simulink library "VANETlib"  (R2019b)
settings: Solver=VariableStepAuto  StartTime=0.0  StopTime=10.0  RelTol=1e-3
PreLoadFcn:
  | vanet_init();
StartFcn:
  | vanet_init();
undefined symbols (not defined in the file or in its folder): fcn_initInfo, m
libraries: $bdroot x2
settings Model: Creator=Le  LastModifiedBy=lewang
settings DataIOCC: ReturnWorkspaceOutputs=off
settings DebuggingCC: ArithmeticOperatorsInVariantConditions=warning
settings SFSimCC: SimUseLocalCustomCode=off  CustomCodeUndefinedFunction=UseInterfaceOnly
settings RTWCC: RTWUseLocalCustomCode=off
settings CodeAppCC: StateflowObjectComments=on

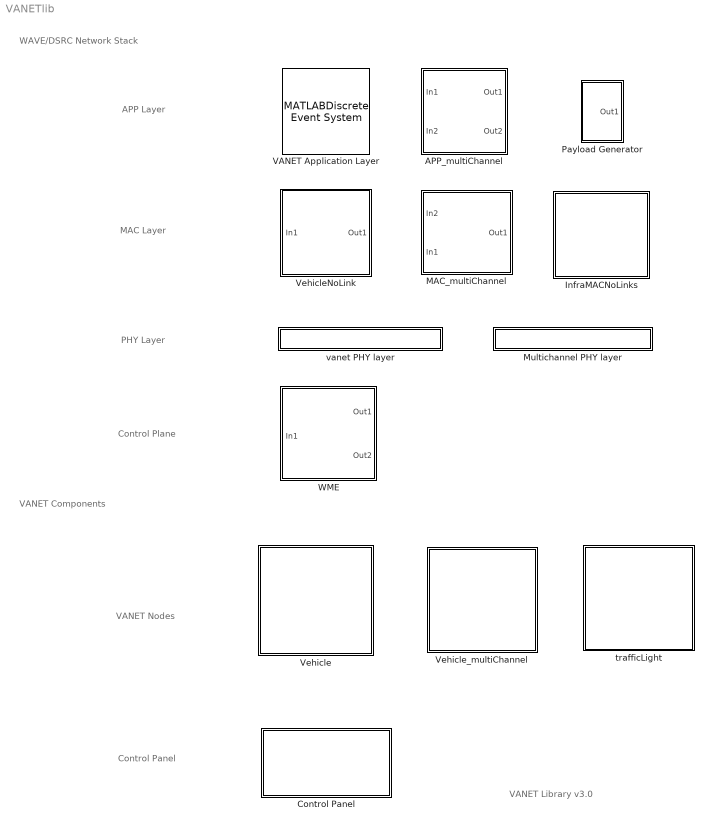
== system VANETlib ==
  note: VANET Components
  note: WAVE/DSRC Network Stack
  note: VANET Library v3.0
  note: APP Layer
  note: MAC Layer
  note: PHY Layer
  note: VANET Nodes
  note: Control Panel
  note: Control Plane
  APP_multiChannel : Subsystem  mask{vehicleID=1, initVelocity=50, initAcc=10, initLane=1, startPositionX=100, startPositionY=0}
      mask prompts: vehicleID "Vehicle ID:"; initVelocity "Start Speed(km/h):"; initAcc "Seconds (0 - 100km/h):"; initLane "Initial Lane (1-4):"; startPositionX "Initial PositionX:"; startPositionY "Initial PositionY:"
      mask Display:
      | str = sprintf('%s\n%s', 'APP', '(Multi-Channel)');
      | disp(str);
  Control Panel : Subsystem  StartFcn=fcn_initInfo('init');  mask{road=highway, roadLength=1600, speedLimit=60, laneChangingOption=Brake without Lane Changing, emgLaneChangingOption=EMG Brake without Lane Changing, txtEnable=off, appTXTEnable=off, isUIon=on, enCCHIext=off}
      mask prompts: road "Road Type"; roadLength "Length of the road (meters)"; speedLimit "Speed limit (km/h)"; laneChangingOption "Lane Changing Option"; emgLaneChangingOption "EMG Lane Changing Option"; txtEnable "Show MAC_PHY Text Process"; appTXTEnable "Show APP Text Process"; isUIon "Graphic UI"; enCCHIext "Enable CCHI_Extension"
      mask init:
      | evalin('base',['txtEnable=' num2str(txtEnable) ';']);
      | evalin('base',['appTXTEnable=' num2str(appTXTEnable) ';']);
      | evalin('base',['roadLength=' num2str(roadLength) ';']);
      | evalin('base',['speedLimit=' num2str(speedLimit) ';']);
      | evalin('base',['isUIon=' num2str(isUIon) ';']);
      | evalin('base',['enCCHIext=' num2str(enCCHIext) ';']);
      mask TypeOptions road: highway | crossRD
      mask Callback road:
      | r=get_param(gcb,'road');
      | assignin('base','road',r);
      mask TypeOptions laneChangingOption: Conservative Lane Changing | Performance Lane Changing | Brake without Lane Changing
      mask Callback laneChangingOption:
      | str=get_param(gcb,'laneChangingOption');
      | 
      | if strcmp(str(1),'C')
      |     assignin('base','brakeMode','ConLaneChange');
      | elseif strcmp(str(1),'P')
      |     assignin('base','brakeMode','PerLaneChange');
      | else
      |     assignin('base','brakeMode','NonLaneChange');
      | end
      mask TypeOptions emgLaneChangingOption: Conservative EMG Lane Changing | Performance EMG Lane Changing | EMG Brake without Lane Changing
      mask Display:
      | str=sprintf('%s\n%s','Parameter','Control Panel');
      | disp(str);
  InfraMACNoLinks : Subsystem
      mask Display:
      | str=sprintf('%s\n%s','InfrastructureMAC','(RoadSideUnit)');
      | disp(str);
  "MAC_multiChannel " : Subsystem  mask{txAddr=0}
      mask prompts: txAddr "Vehicle ID"
      mask Display:
      | str = sprintf('%s\n%s', 'VehicleMAC','(Multi-Channel)');
      | disp(str);
  Multichannel PHY layer : Subsystem  mask{numStations=4}
      mask prompts: numStations "Number of vehicles"
      mask init:
      | evalin('base',['numStations=' num2str(numStations) ';']);
      mask Display: disp('Wireless MultiChannel');
  Payload Generator : Subsystem  mask{txAddr=1, ac0Rate=1, ac1Rate=1, ac2Rate=1, ac3Rate=1}
      mask prompts: txAddr "StationID"; ac0Rate "AC0"; ac1Rate "AC1"; ac2Rate "AC2"; ac3Rate "AC3"
      mask Display: disp('msg');
  VANET Application Layer : MATLABDiscreteEventSystem  InputPortMessageModes=m  OutputPortMessageModes=m  System=des_APP_OBU  vehicleID=1  initVelocity=10  initAcc=10  initLane=1  startPositionX=10  startPositionY=0  SimulateUsing=Code generation
      mask Type: des_APP_OBU
      mask Display: disp('des_APP_OBU');
  Vehicle : Subsystem  mask{carID=1, startSpd=50, startAcc=10, initLane=1, startPosX=0, startPosY=0}
      mask prompts: carID "VehilcleID"; startSpd "Initial Speed (Km/h):"; startAcc "Seconds from 0 - 100 Km/h:"; initLane "Initial lane number (1-4) :"; startPosX "Initial PositionX"; startPosY "Initial PositionY"
      mask Display:
      | str=sprintf('%s\n%s','Vehicle','(APP-MAC-PHY)');
      | disp(str);
      | 
      | image('figs/car2.jpg');
  VehicleNoLink : Subsystem  mask{txAddr=1, V2x=V2V, infraAddress=0, Retry_MAX=3, AC0=9, AC1=6, AC2=3, AC3=2, aCWmin=15, aCWmax=1023, slottime=13, SIFS=32}
      mask prompts: txAddr "Vehicle ID"; V2x "V2X Mode"; infraAddress "AP"; Retry_MAX "Max Retransmissions (3-8):"; AC0 "AIFSN(AC0):"; AC1 "AIFSN(AC1):"; AC2 "AIFSN(AC2):"; AC3 "AIFSN(AC3):"; slottime "slotTime (us):"; SIFS "SIFS (us):"
      mask TypeOptions V2x: V2V | V2I
      mask Callback V2x:
      | V2Xmode=get_param(gcb,'V2x');
      | 
      | if strcmp(V2Xmode,'V2V')
      |     set_param(gcb,'MaskVisibilities',{'on';'on';'off';'on';'on';'on';'on';'on';'on';'on';'on';'on'});
      | 
      | elseif strcmp(V2Xmode,'V2I')
      |     set_param(gcb,'MaskVisibilities',{'on';'on';'on';'on';'on';'on';'on';'on';'on';'on';'on';'on'});
      | end
      mask DialogControl netParams Prompt: Network Parameters
      mask DialogControl Basic Prompt: Basic Information
      mask DialogControl EDCA Prompt: EDCA Parameter
      mask Display:
      | str=sprintf('%s\n%s','VehicleMAC','(OnBoardUnit)');
      | disp(str);
  Vehicle_multiChannel : Subsystem  mask{vehicleID=1, startSpd=50, startAcc=10, initLane=1, startPosX=100, startPosY=0, MCsvcRole=Service User}
      mask prompts: vehicleID "Vehicle ID"; startSpd "Initial Speed(km/h):"; startAcc "Seconds from 0-100 km/h:"; initLane "Initial lane number(1-4):"; startPosX "Initial PositionX:"; startPosY "Initial PositionY:"; MCsvcRole "Service Role (Provider/User):"
      mask TypeOptions MCsvcRole: Service Provider | Service User
      mask Callback MCsvcRole: MCsvcRole=get_param(gcb,'MCsvcRole');
      mask Display:
      | %disp('vehicle_multiChan');
      | 
      | image('figs/car2.png');
  WME : Subsystem  mask{vehicleID=1}
      mask prompts: vehicleID "Vehicle ID"
      mask Display:
      | str = sprintf('%s\n\n%s\n\n%s\n\n%s', 'WAVE', 'Management', 'Entity', '(WME)');
      | disp(str);
  trafficLight : Subsystem  mask{green=26, yellow=4}
      mask prompts: green "Green Light Duration"; yellow "Yellow Light Duration"
      mask Display:
      | str=sprintf('%s','Traffic Light');
      | disp(str);
      | 
      | image('figs/light2.jpg');
  vanet PHY layer : Subsystem  mask{numStations=0}
      mask prompts: numStations "Number of Vehicles"
      mask init:
      | evalin('base',['numStations=' num2str(numStations) ';']);
      mask Display:
      | disp('Wireless Channel');
      | % image('figs/wave1.png');

== system VANETlib/APP_multiChannel ==
  In1 : Inport
  In2 : Inport  Port=2
  MATLAB Discrete-Event System : MATLABDiscreteEventSystem  InputPortMessageModes=m,m  OutputPortMessageModes=m,m  System=des_APP_mulChan_OBU  vehicleID=vehicleID  initVelocity=initVelocity  initAcc=initAcc  initLane=initLane  startPositionX=startPositionX  startPositionY=startPositionY  svcRole=0  SimulateUsing=Code generation
      mask Type: des_APP_mulChan_OBU
      mask Display: disp('des_APP_mulChan_OBU');
  Out1 : Outport  VectorParamsAs1DForOutWhenUnconnected=off
  Out2 : Outport  Port=2  VectorParamsAs1DForOutWhenUnconnected=off
  wires:
  MATLAB Discrete-Event System/2 -> Out2/1
  In1/1 -> MATLAB Discrete-Event System/1
  In2/1 -> MATLAB Discrete-Event System/2
  MATLAB Discrete-Event System/1 -> Out1/1

== system VANETlib/Control Panel ==

== system VANETlib/InfraMACNoLinks ==
  Entity Multicast : EntityMulticast  InputPortMessageModes=m  MulticastTag=toPhy
  MATLAB Discrete-Event System : MATLABDiscreteEventSystem  InputPortMessageModes=m  OutputPortMessageModes=m  System=des_MAC_RSU  Retry_MAX=3  AIFSN_AC0=9  AIFSN_AC1=6  AIFSN_AC2=3  AIFSN_AC3=2  aCWmin=15  aCWmax=1023  slottime=0.000013  sifs=0.000032  propTime=1  BSSID=00  rxAddr=0  SimulateUsing=Code generation
      mask Type: des_MAC_RSU
      mask Display: disp('des_MAC_RSU');
  Multicast Receive Queue : Queue  OutputPortMessageModes=m  Capacity=inf  EntityArrivalSource=Multicast  MulticastTag=fromPhy
  wires:
  Multicast Receive Queue/1 -> MATLAB Discrete-Event System/1
  MATLAB Discrete-Event System/1 -> Entity Multicast/1

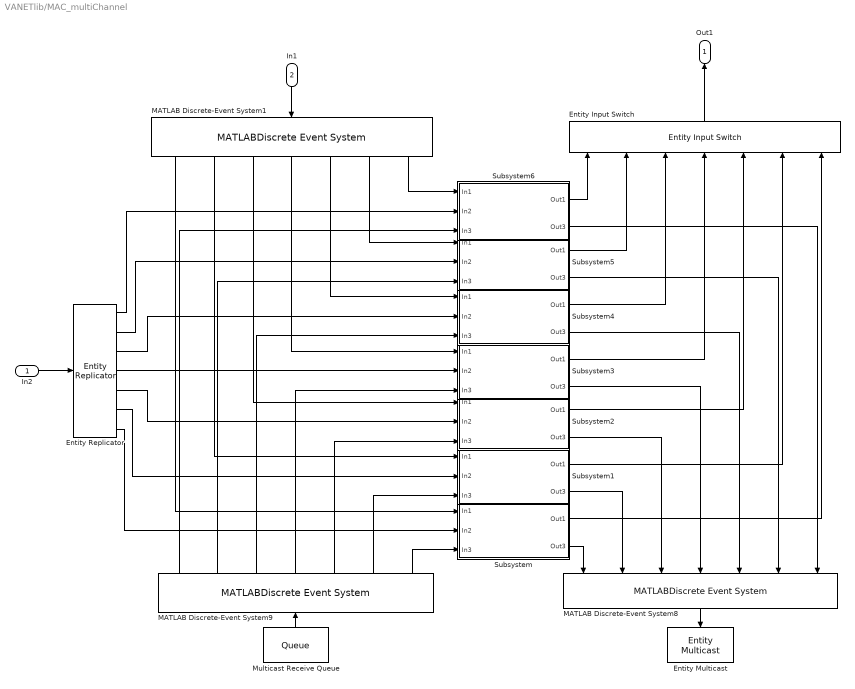
== system VANETlib/MAC_multiChannel  ==
  In2 : Inport
  In1 : Inport  Port=2
  Entity Input Switch : EntityInputSwitch  InputPortMessageModes=m,m,m,m,m,m,m  OutputPortMessageModes=m  NumberInputPorts=7  SwitchingCriterion=Equiprobable
      settings: InputPortMap=u1,u2,u3,u4,u5,u6,u7
  Entity Multicast : EntityMulticast  InputPortMessageModes=m  MulticastTag=toPhy
  Entity Replicator : EntityReplicator  InputPortMessageModes=m  OutputPortMessageModes=m,m,m,m,m,m,m  NumberReplicas=6
      settings: OutputPortMap=o0,o1,o2,o3,o4,o5,o6
  MATLAB Discrete-Event System1 : MATLABDiscreteEventSystem  InputPortMessageModes=m  OutputPortMessageModes=m,m,m,m,m,m,m  System=des_MAC_channelRouting  SimulateUsing=Code generation
      mask Type: des_MAC_channelRouting
      mask Display: disp('des_MAC_channelRouting');
  MATLAB Discrete-Event System8 : MATLABDiscreteEventSystem  InputPortMessageModes=m,m,m,m,m,m,m  OutputPortMessageModes=m  System=des_MAC_channelSelect  SimulateUsing=Code generation
      mask Type: des_MAC_channelSelect
      mask Display: disp('des_MAC_channelSelect');
  MATLAB Discrete-Event System9 : MATLABDiscreteEventSystem  InputPortMessageModes=m  OutputPortMessageModes=m,m,m,m,m,m,m  System=des_MAC_macSelect  SimulateUsing=Code generation
      mask Type: des_MAC_macSelect
      mask Display: disp('des_MAC_macSelect');
  Multicast Receive Queue : Queue  OutputPortMessageModes=m  Capacity=inf  EntityArrivalSource=Multicast  MulticastTag=fromPhy
  Subsystem : Subsystem  mask{chanNum=0}
      mask prompts: chanNum "Channel Number (CCH - 0) :"
      mask Display: disp('CCH - 0');
  Subsystem1 : Subsystem  mask{chanNum=1}
      mask prompts: chanNum "Channel Num (SCH (1-6)):"
      mask Display: disp('SCH - 1');
  Subsystem2 : Subsystem  mask{chanNum=2}
      mask prompts: chanNum "Channel Number (SCH (1-6)) :"
      mask Display: disp('SCH - 2');
  Subsystem3 : Subsystem  mask{chanNum=3}
      mask prompts: chanNum "Channel Number (SCH (1-6)):"
      mask Display: disp('SCH - 3');
  Subsystem4 : Subsystem  mask{chanNum=4}
      mask prompts: chanNum "Channel Number (SCH (1-6)):"
      mask Display: disp('SCH - 4');
  Subsystem5 : Subsystem  mask{chanNum=5}
      mask prompts: chanNum "Channel Number (SCH (1-6)):"
      mask Display: disp('SCH - 5');
  Subsystem6 : Subsystem  mask{chanNum=6}
      mask prompts: chanNum "Channel Number (SCH (1-6)):"
      mask Display: disp('SCH - 6');
  Out1 : Outport  VectorParamsAs1DForOutWhenUnconnected=off
  wires:
  Subsystem3/2(Out3) -> MATLAB Discrete-Event System8/4
  Entity Replicator/7 -> Subsystem/2(In2)
  Subsystem5/2(Out3) -> MATLAB Discrete-Event System8/6
  MATLAB Discrete-Event System9/7 -> Subsystem/3(In3)
  Entity Replicator/5 -> Subsystem2/2(In2)
  MATLAB Discrete-Event System1/7 -> Subsystem6/1(In1)
  Entity Replicator/4 -> Subsystem3/2(In2)
  MATLAB Discrete-Event System1/3 -> Subsystem2/1(In1)
  Subsystem6/1(Out1) -> Entity Input Switch/1
  MATLAB Discrete-Event System9/4 -> Subsystem3/3(In3)
  Subsystem4/2(Out3) -> MATLAB Discrete-Event System8/5
  MATLAB Discrete-Event System9/6 -> Subsystem1/3(In3)
  Subsystem1/2(Out3) -> MATLAB Discrete-Event System8/2
  MATLAB Discrete-Event System1/1 -> Subsystem/1(In1)
  Subsystem/1(Out1) -> Entity Input Switch/7
  Entity Replicator/3 -> Subsystem4/2(In2)
  MATLAB Discrete-Event System9/1 -> Subsystem6/3(In3)
  In2/1 -> Entity Replicator/1
  MATLAB Discrete-Event System1/6 -> Subsystem5/1(In1)
  Subsystem2/2(Out3) -> MATLAB Discrete-Event System8/3
  MATLAB Discrete-Event System8/1 -> Entity Multicast/1
  MATLAB Discrete-Event System9/5 -> Subsystem2/3(In3)
  MATLAB Discrete-Event System9/2 -> Subsystem5/3(In3)
  Subsystem3/1(Out1) -> Entity Input Switch/4
  Subsystem2/1(Out1) -> Entity Input Switch/5
  MATLAB Discrete-Event System9/3 -> Subsystem4/3(In3)
  Subsystem5/1(Out1) -> Entity Input Switch/2
  Entity Input Switch/1 -> Out1/1
  Subsystem1/1(Out1) -> Entity Input Switch/6
  MATLAB Discrete-Event System1/2 -> Subsystem1/1(In1)
  Subsystem6/2(Out3) -> MATLAB Discrete-Event System8/7
  MATLAB Discrete-Event System1/4 -> Subsystem3/1(In1)
  In1/1 -> MATLAB Discrete-Event System1/1
  MATLAB Discrete-Event System1/5 -> Subsystem4/1(In1)
  Subsystem4/1(Out1) -> Entity Input Switch/3
  Entity Replicator/2 -> Subsystem5/2(In2)
  Subsystem/2(Out3) -> MATLAB Discrete-Event System8/1
  Multicast Receive Queue/1 -> MATLAB Discrete-Event System9/1
  Entity Replicator/6 -> Subsystem1/2(In2)
  Entity Replicator/1 -> Subsystem6/2(In2)

== system VANETlib/Multichannel PHY layer ==
  Entity Multicast2 : EntityMulticast  InputPortMessageModes=m  MulticastTag=fromPhy
  MATLAB Discrete-Event System : MATLABDiscreteEventSystem  InputPortMessageModes=m  OutputPortMessageModes=m  System=des_PHY_mulChan_links  SimulateUsing=Code generation
      mask Type: des_PHY_mulChan_links
      mask Display: disp('des_PHY_mulChan_links');
  Multicast Receive Queue2 : Queue  OutputPortMessageModes=m  Capacity=inf  EntityArrivalSource=Multicast  MulticastTag=toPhy
  wires:
  Multicast Receive Queue2/1 -> MATLAB Discrete-Event System/1
  MATLAB Discrete-Event System/1 -> Entity Multicast2/1

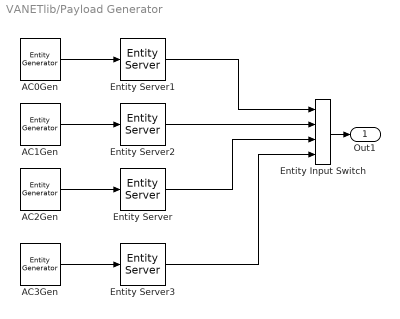
== system VANETlib/Payload Generator ==
  AC0Gen : EntityGenerator  OutputPortMessageModes=m  TimeSource=MATLAB action  Period=0.1  IntergenerationTimeAction=|  GenerateEntityAtSimulationStart=off  GenerateAction=|  EntityType=Bus object  EntityTypeName=Payload
      IntergenerationTimeAction=|
      | % y=getParams();
      | dt=ac0Rate;
      GenerateAction=|
      | coder.extrinsic('evalin')
      | payloadlength=evalin('base','payloadLength');
      | entity.wsmp=ones(1,payloadlength);
      | % rng('shuffle');
      | entity.priority=1;
  AC1Gen : EntityGenerator  OutputPortMessageModes=m  TimeSource=MATLAB action  Period=0.1  IntergenerationTimeAction=|  GenerateEntityAtSimulationStart=off  GenerateAction=|  EntityType=Bus object  EntityTypeName=Payload
      IntergenerationTimeAction=|
      | % y=getParams();
      | dt=ac1Rate;
      GenerateAction=|
      | coder.extrinsic('evalin')
      | payloadlength=evalin('base','payloadLength');
      | entity.wsmp=ones(1,payloadlength);
      | % rng('shuffle');
      | entity.priority=3;
  AC2Gen : EntityGenerator  OutputPortMessageModes=m  TimeSource=MATLAB action  Period=0.1  IntergenerationTimeAction=|  GenerateEntityAtSimulationStart=off  GenerateAction=|  EntityType=Bus object  EntityTypeName=Payload
      IntergenerationTimeAction=|
      | % y=getParams();
      | dt=ac2Rate;
      GenerateAction=|
      | coder.extrinsic('evalin')
      | payloadlength=evalin('base','payloadLength');
      | entity.wsmp=ones(1,payloadlength);
      | entity.VehicleID=txAddr;
      | % rng('shuffle');
      | entity.priority=5;
  AC3Gen : EntityGenerator  OutputPortMessageModes=m  TimeSource=MATLAB action  Period=0.1  IntergenerationTimeAction=|  GenerateEntityAtSimulationStart=off  GenerateAction=|  EntityType=Bus object  EntityTypeName=Payload
      IntergenerationTimeAction=|
      | % dt=exponentialArrivalTime();
      | dt=ac3Rate;
      GenerateAction=|
      | coder.extrinsic('evalin')
      | payloadLength=evalin('base','payloadLength');
      | entity.wsmp=ones(1,payloadLength);
      | 
      | % entity.wsmp=msg2wsmp(txAddr,entity.wsmp,1);
      | % rng('shuffle');
      | entity.priority=7;
  Entity Input Switch : EntityInputSwitch  InputPortMessageModes=m,m,m,m  OutputPortMessageModes=m  NumberInputPorts=4
      settings: InputPortMap=u1,u2,u3,u4
  Entity Server : EntityServer  InputPortMessageModes=m  OutputPortMessageModes=m  Capacity=1  ServiceTimeSource=MATLAB action  ServiceTimeAction=dt = 0.000002*txAddr;
  Entity Server1 : EntityServer  InputPortMessageModes=m  OutputPortMessageModes=m  Capacity=1  ServiceTimeSource=MATLAB action  ServiceTimeAction=dt = 0.000004*txAddr;
  Entity Server2 : EntityServer  InputPortMessageModes=m  OutputPortMessageModes=m  Capacity=1  ServiceTimeSource=MATLAB action  ServiceTimeAction=dt = 0.000003*txAddr;
  Entity Server3 : EntityServer  InputPortMessageModes=m  OutputPortMessageModes=m  Capacity=1  ServiceTimeSource=MATLAB action  ServiceTimeAction=dt = 0.000001*txAddr;
  Out1 : Outport  VectorParamsAs1DForOutWhenUnconnected=off
  wires:
  AC2Gen/1 -> Entity Server/1
  Entity Server/1 -> Entity Input Switch/3
  Entity Input Switch/1 -> Out1/1
  AC0Gen/1 -> Entity Server1/1
  Entity Server1/1 -> Entity Input Switch/1
  AC1Gen/1 -> Entity Server2/1
  Entity Server2/1 -> Entity Input Switch/2
  AC3Gen/1 -> Entity Server3/1
  Entity Server3/1 -> Entity Input Switch/4

== system VANETlib/Vehicle ==
  VANET Application Layer1 : $bdroot/VANET Application Layer  vehicleID=carID  initVelocity=startSpd  initAcc=startAcc  initLane=initLane  startPositionX=startPosX  startPositionY=startPosY  SimulateUsing=Code generation
  VehicleOI1 : $bdroot/VehicleNoLink  txAddr=carID  V2x=V2V  infraAddress=0  Retry_MAX=3  AC0=9  AC1=6  AC2=3  AC3=2  aCWmin=15  aCWmax=1023  slottime=13  SIFS=32
  wires:
  VehicleOI1/1 -> VANET Application Layer1/1
  VANET Application Layer1/1 -> VehicleOI1/1

== system VANETlib/VehicleNoLink ==
  In1 : Inport
  Entity Multicast : EntityMulticast  InputPortMessageModes=m  MulticastTag=toPhy
  Multicast Receive Queue : Queue  OutputPortMessageModes=m  Capacity=inf  EntityArrivalSource=Multicast  MulticastTag=fromPhy
  vehicular OBU : MATLABDiscreteEventSystem  InputPortMessageModes=m,m  OutputPortMessageModes=m,m  System=des_MAC_OBU  Retry_MAX=Retry_MAX  AIFSN_AC0=AC0  AIFSN_AC1=AC1  AIFSN_AC2=AC2  AIFSN_AC3=AC3  aCWmin=aCWmin  aCWmax=aCWmax  slottime=slottime  sifs=SIFS  txAddr=txAddr  infraAddress=infraAddress  SimulateUsing=Code generation
      mask Type: des_MAC_OBU
      mask Display: disp('des_MAC_OBU');
  Out1 : Outport  VectorParamsAs1DForOutWhenUnconnected=off
  wires:
  In1/1 -> vehicular OBU/1
  vehicular OBU/1 -> Out1/1
  Multicast Receive Queue/1 -> vehicular OBU/2
  vehicular OBU/2 -> Entity Multicast/1

== system VANETlib/Vehicle_multiChannel ==
  MATLAB Discrete-Event System1 : MATLABDiscreteEventSystem  InputPortMessageModes=m,m  OutputPortMessageModes=m,m  System=des_APP_mulChan_OBU  vehicleID=vehicleID  initVelocity=startSpd  initAcc=startAcc  initLane=initLane  startPositionX=startPosX  startPositionY=startPosY  svcRole=0  SimulateUsing=Code generation
      mask Type: des_APP_mulChan_OBU
      mask Display: disp('des_APP_mulChan_OBU');
  Subsystem1 : Subsystem  mask{txAddr=vehicleID}
      mask prompts: txAddr "Vehicle ID"
      mask Display: disp('des_MAC_mulChan_OBU');
  Subsystem2 : Subsystem  mask{vehicleID=vehicleID}
      mask prompts: vehicleID "Vehicle ID"
      mask Display:
      | str = sprintf('%s\n\n%s\n\n%s\n\n%s', 'WAVE', 'Management', 'Entity', '(WME)');
      | disp(str);
  wires:
  Subsystem2/2(Out2) -> Subsystem1/1(In2)
  MATLAB Discrete-Event System1/1 -> Subsystem1/2(In1)
  Subsystem1/1(Out1) -> MATLAB Discrete-Event System1/1
  Subsystem2/1(Out1) -> MATLAB Discrete-Event System1/2
  MATLAB Discrete-Event System1/2 -> Subsystem2/1(In1)

== system VANETlib/WME ==
  In1 : Inport
  MATLAB Discrete-Event System : MATLABDiscreteEventSystem  InputPortMessageModes=m  OutputPortMessageModes=m,m  System=des_APP_WME  vehicleID=0  enCCHIext=0  SimulateUsing=Code generation
      mask Type: des_APP_WME
      mask Display: disp('des_APP_WME');
  Out1 : Outport  VectorParamsAs1DForOutWhenUnconnected=off
  Out2 : Outport  Port=2  VectorParamsAs1DForOutWhenUnconnected=off
  wires:
  MATLAB Discrete-Event System/1 -> Out1/1
  In1/1 -> MATLAB Discrete-Event System/1
  MATLAB Discrete-Event System/2 -> Out2/1

== system VANETlib/trafficLight ==
  Entity Generator : EntityGenerator  OutputPortMessageModes=m  Period=inf  GenerateAction=|  AttributeName=entity  AttributeInitialValue=0  EntityTypeName=Entity
      | persistent n
      | if isempty(n)
      |     n=1;
      | end
      | 
      | entity=n;
      | n=n+1;
  Entity Terminator : EntityTerminator  InputPortMessageModes=m
  MATLAB Discrete-Event System : MATLABDiscreteEventSystem  InputPortMessageModes=m  OutputPortMessageModes=m  System=des_trafficlight  greenLight=green  yellowLight=yellow  SimulateUsing=Code generation
      mask Type: des_trafficlight
      mask Display: disp('des_trafficlight');
  wires:
  MATLAB Discrete-Event System/1 -> Entity Terminator/1
  Entity Generator/1 -> MATLAB Discrete-Event System/1

== system VANETlib/vanet PHY layer ==
  Entity Multicast2 : EntityMulticast  InputPortMessageModes=m  MulticastTag=fromPhy
  Multicast Receive Queue2 : Queue  OutputPortMessageModes=m  Capacity=inf  EntityArrivalSource=Multicast  MulticastTag=toPhy
  V2x Links : MATLABDiscreteEventSystem  InputPortMessageModes=m  OutputPortMessageModes=m  System=des_PHY_links  SimulateUsing=Code generation
      mask Type: des_PHY_links
      mask Display: disp('des_PHY_links');
  wires:
  V2x Links/1 -> Entity Multicast2/1
  Multicast Receive Queue2/1 -> V2x Links/1

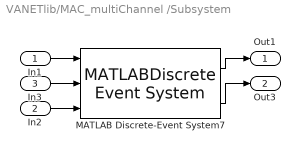
== system VANETlib/MAC_multiChannel /Subsystem ==
  In1 : Inport
  In2 : Inport  Port=2
  In3 : Inport  Port=3
  MATLAB Discrete-Event System7 : MATLABDiscreteEventSystem  InputPortMessageModes=m,m,m  OutputPortMessageModes=m,m  System=des_MAC_mulChan_OBU  Retry_MAX=3  AIFSN_AC0=9  AIFSN_AC1=6  AIFSN_AC2=3  AIFSN_AC3=2  aCWmin=15  aCWmax=1023  slottime=13  sifs=32  txAddr=txAddr  infraAddress=0  ChanNum=chanNum  SimulateUsing=Code generation
      mask Type: des_MAC_mulChan_OBU
      mask Display: disp('des_MAC_mulChan_OBU');
  Out1 : Outport  VectorParamsAs1DForOutWhenUnconnected=off
  Out3 : Outport  Port=2  VectorParamsAs1DForOutWhenUnconnected=off
  wires:
  In1/1 -> MATLAB Discrete-Event System7/1
  MATLAB Discrete-Event System7/2 -> Out3/1
  MATLAB Discrete-Event System7/1 -> Out1/1
  In3/1 -> MATLAB Discrete-Event System7/2
  In2/1 -> MATLAB Discrete-Event System7/3

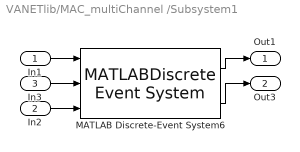
== system VANETlib/MAC_multiChannel /Subsystem1 ==
  In1 : Inport
  In2 : Inport  Port=2
  In3 : Inport  Port=3
  MATLAB Discrete-Event System6 : MATLABDiscreteEventSystem  InputPortMessageModes=m,m,m  OutputPortMessageModes=m,m  System=des_MAC_mulChan_OBU  Retry_MAX=3  AIFSN_AC0=9  AIFSN_AC1=6  AIFSN_AC2=3  AIFSN_AC3=2  aCWmin=15  aCWmax=1023  slottime=13  sifs=32  txAddr=txAddr  infraAddress=0  ChanNum=chanNum  SimulateUsing=Code generation
      mask Type: des_MAC_mulChan_OBU
      mask Display: disp('des_MAC_mulChan_OBU');
  Out1 : Outport  VectorParamsAs1DForOutWhenUnconnected=off
  Out3 : Outport  Port=2  VectorParamsAs1DForOutWhenUnconnected=off
  wires:
  In2/1 -> MATLAB Discrete-Event System6/3
  MATLAB Discrete-Event System6/1 -> Out1/1
  In1/1 -> MATLAB Discrete-Event System6/1
  MATLAB Discrete-Event System6/2 -> Out3/1
  In3/1 -> MATLAB Discrete-Event System6/2

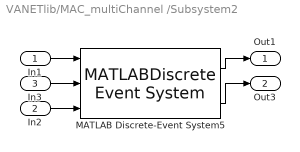
== system VANETlib/MAC_multiChannel /Subsystem2 ==
  In1 : Inport
  In2 : Inport  Port=2
  In3 : Inport  Port=3
  MATLAB Discrete-Event System5 : MATLABDiscreteEventSystem  InputPortMessageModes=m,m,m  OutputPortMessageModes=m,m  System=des_MAC_mulChan_OBU  Retry_MAX=3  AIFSN_AC0=9  AIFSN_AC1=6  AIFSN_AC2=3  AIFSN_AC3=2  aCWmin=15  aCWmax=1023  slottime=13  sifs=32  txAddr=txAddr  infraAddress=0  ChanNum=chanNum  SimulateUsing=Code generation
      mask Type: des_MAC_mulChan_OBU
      mask Display: disp('des_MAC_mulChan_OBU');
  Out1 : Outport  VectorParamsAs1DForOutWhenUnconnected=off
  Out3 : Outport  Port=2  VectorParamsAs1DForOutWhenUnconnected=off
  wires:
  In2/1 -> MATLAB Discrete-Event System5/3
  MATLAB Discrete-Event System5/1 -> Out1/1
  In3/1 -> MATLAB Discrete-Event System5/2
  MATLAB Discrete-Event System5/2 -> Out3/1
  In1/1 -> MATLAB Discrete-Event System5/1

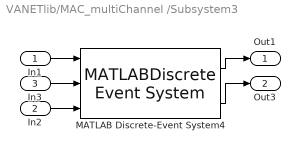
== system VANETlib/MAC_multiChannel /Subsystem3 ==
  In1 : Inport
  In2 : Inport  Port=2
  In3 : Inport  Port=3
  MATLAB Discrete-Event System4 : MATLABDiscreteEventSystem  InputPortMessageModes=m,m,m  OutputPortMessageModes=m,m  System=des_MAC_mulChan_OBU  Retry_MAX=3  AIFSN_AC0=9  AIFSN_AC1=6  AIFSN_AC2=3  AIFSN_AC3=2  aCWmin=15  aCWmax=1023  slottime=13  sifs=32  txAddr=txAddr  infraAddress=0  ChanNum=chanNum  SimulateUsing=Code generation
      mask Type: des_MAC_mulChan_OBU
      mask Display: disp('des_MAC_mulChan_OBU');
  Out1 : Outport  VectorParamsAs1DForOutWhenUnconnected=off
  Out3 : Outport  Port=2  VectorParamsAs1DForOutWhenUnconnected=off
  wires:
  In2/1 -> MATLAB Discrete-Event System4/3
  In3/1 -> MATLAB Discrete-Event System4/2
  In1/1 -> MATLAB Discrete-Event System4/1
  MATLAB Discrete-Event System4/2 -> Out3/1
  MATLAB Discrete-Event System4/1 -> Out1/1

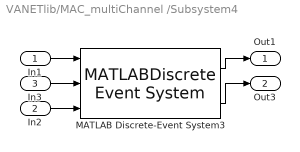
== system VANETlib/MAC_multiChannel /Subsystem4 ==
  In1 : Inport
  In2 : Inport  Port=2
  In3 : Inport  Port=3
  MATLAB Discrete-Event System3 : MATLABDiscreteEventSystem  InputPortMessageModes=m,m,m  OutputPortMessageModes=m,m  System=des_MAC_mulChan_OBU  Retry_MAX=3  AIFSN_AC0=9  AIFSN_AC1=6  AIFSN_AC2=3  AIFSN_AC3=2  aCWmin=15  aCWmax=1023  slottime=13  sifs=32  txAddr=txAddr  infraAddress=0  ChanNum=chanNum  SimulateUsing=Code generation
      mask Type: des_MAC_mulChan_OBU
      mask Display: disp('des_MAC_mulChan_OBU');
  Out1 : Outport  VectorParamsAs1DForOutWhenUnconnected=off
  Out3 : Outport  Port=2  VectorParamsAs1DForOutWhenUnconnected=off
  wires:
  MATLAB Discrete-Event System3/2 -> Out3/1
  In1/1 -> MATLAB Discrete-Event System3/1
  MATLAB Discrete-Event System3/1 -> Out1/1
  In2/1 -> MATLAB Discrete-Event System3/3
  In3/1 -> MATLAB Discrete-Event System3/2

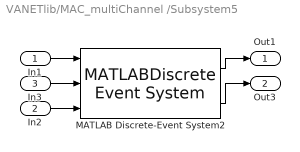
== system VANETlib/MAC_multiChannel /Subsystem5 ==
  In1 : Inport
  In2 : Inport  Port=2
  In3 : Inport  Port=3
  MATLAB Discrete-Event System2 : MATLABDiscreteEventSystem  InputPortMessageModes=m,m,m  OutputPortMessageModes=m,m  System=des_MAC_mulChan_OBU  Retry_MAX=3  AIFSN_AC0=9  AIFSN_AC1=6  AIFSN_AC2=3  AIFSN_AC3=2  aCWmin=15  aCWmax=1023  slottime=13  sifs=32  txAddr=txAddr  infraAddress=0  ChanNum=chanNum  SimulateUsing=Code generation
      mask Type: des_MAC_mulChan_OBU
      mask Display: disp('des_MAC_mulChan_OBU');
  Out1 : Outport  VectorParamsAs1DForOutWhenUnconnected=off
  Out3 : Outport  Port=2  VectorParamsAs1DForOutWhenUnconnected=off
  wires:
  In1/1 -> MATLAB Discrete-Event System2/1
  MATLAB Discrete-Event System2/1 -> Out1/1
  In3/1 -> MATLAB Discrete-Event System2/2
  In2/1 -> MATLAB Discrete-Event System2/3
  MATLAB Discrete-Event System2/2 -> Out3/1

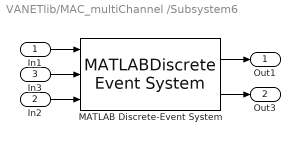
== system VANETlib/MAC_multiChannel /Subsystem6 ==
  In1 : Inport
  In2 : Inport  Port=2
  In3 : Inport  Port=3
  MATLAB Discrete-Event System : MATLABDiscreteEventSystem  InputPortMessageModes=m,m,m  OutputPortMessageModes=m,m  System=des_MAC_mulChan_OBU  Retry_MAX=3  AIFSN_AC0=9  AIFSN_AC1=6  AIFSN_AC2=3  AIFSN_AC3=2  aCWmin=15  aCWmax=1023  slottime=13  sifs=32  txAddr=txAddr  infraAddress=0  ChanNum=chanNum  SimulateUsing=Code generation
      mask Type: des_MAC_mulChan_OBU
      mask Display: disp('des_MAC_mulChan_OBU');
  Out1 : Outport  VectorParamsAs1DForOutWhenUnconnected=off
  Out3 : Outport  Port=2  VectorParamsAs1DForOutWhenUnconnected=off
  wires:
  MATLAB Discrete-Event System/1 -> Out1/1
  In2/1 -> MATLAB Discrete-Event System/3
  In1/1 -> MATLAB Discrete-Event System/1
  In3/1 -> MATLAB Discrete-Event System/2
  MATLAB Discrete-Event System/2 -> Out3/1

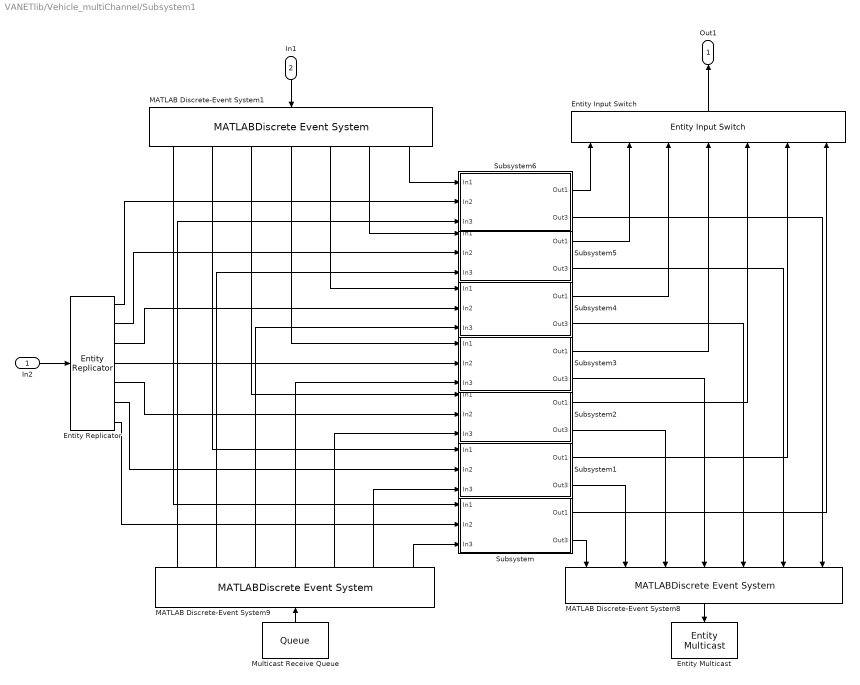
== system VANETlib/Vehicle_multiChannel/Subsystem1 ==
  In2 : Inport
  In1 : Inport  Port=2
  Entity Input Switch : EntityInputSwitch  InputPortMessageModes=m,m,m,m,m,m,m  OutputPortMessageModes=m  NumberInputPorts=7  SwitchingCriterion=Equiprobable
      settings: InputPortMap=u1,u2,u3,u4,u5,u6,u7
  Entity Multicast : EntityMulticast  InputPortMessageModes=m  MulticastTag=toPhy
  Entity Replicator : EntityReplicator  InputPortMessageModes=m  OutputPortMessageModes=m,m,m,m,m,m,m  NumberReplicas=6
      settings: OutputPortMap=o0,o1,o2,o3,o4,o5,o6
  MATLAB Discrete-Event System1 : MATLABDiscreteEventSystem  InputPortMessageModes=m  OutputPortMessageModes=m,m,m,m,m,m,m  System=des_MAC_channelRouting  SimulateUsing=Code generation
      mask Type: des_MAC_channelRouting
      mask Display: disp('des_MAC_channelRouting');
  MATLAB Discrete-Event System8 : MATLABDiscreteEventSystem  InputPortMessageModes=m,m,m,m,m,m,m  OutputPortMessageModes=m  System=des_MAC_channelSelect  SimulateUsing=Code generation
      mask Type: des_MAC_channelSelect
      mask Display: disp('des_MAC_channelSelect');
  MATLAB Discrete-Event System9 : MATLABDiscreteEventSystem  InputPortMessageModes=m  OutputPortMessageModes=m,m,m,m,m,m,m  System=des_MAC_macSelect  SimulateUsing=Code generation
      mask Type: des_MAC_macSelect
      mask Display: disp('des_MAC_macSelect');
  Multicast Receive Queue : Queue  OutputPortMessageModes=m  Capacity=inf  EntityArrivalSource=Multicast  MulticastTag=fromPhy
  Subsystem : Subsystem  mask{chanNum=0}
      mask prompts: chanNum "Channel Number (CCH - 0) :"
      mask Display: disp('CCH - 0');
  Subsystem1 : Subsystem  mask{chanNum=1}
      mask prompts: chanNum "Channel Num (SCH (1-6)):"
      mask Display: disp('SCH - 1');
  Subsystem2 : Subsystem  mask{chanNum=2}
      mask prompts: chanNum "Channel Number (SCH (1-6)) :"
      mask Display: disp('SCH - 2');
  Subsystem3 : Subsystem  mask{chanNum=3}
      mask prompts: chanNum "Channel Number (SCH (1-6)):"
      mask Display: disp('SCH - 3');
  Subsystem4 : Subsystem  mask{chanNum=4}
      mask prompts: chanNum "Channel Number (SCH (1-6)):"
      mask Display: disp('SCH - 4');
  Subsystem5 : Subsystem  mask{chanNum=5}
      mask prompts: chanNum "Channel Number (SCH (1-6)):"
      mask Display: disp('SCH - 5');
  Subsystem6 : Subsystem  mask{chanNum=6}
      mask prompts: chanNum "Channel Number (SCH (1-6)):"
      mask Display: disp('SCH - 6');
  Out1 : Outport  VectorParamsAs1DForOutWhenUnconnected=off
  wires:
  MATLAB Discrete-Event System1/7 -> Subsystem6/1(In1)
  MATLAB Discrete-Event System9/6 -> Subsystem1/3(In3)
  MATLAB Discrete-Event System9/2 -> Subsystem5/3(In3)
  MATLAB Discrete-Event System8/1 -> Entity Multicast/1
  Subsystem5/1(Out1) -> Entity Input Switch/2
  Subsystem5/2(Out3) -> MATLAB Discrete-Event System8/6
  Subsystem6/1(Out1) -> Entity Input Switch/1
  Subsystem1/2(Out3) -> MATLAB Discrete-Event System8/2
  Subsystem6/2(Out3) -> MATLAB Discrete-Event System8/7
  Subsystem/1(Out1) -> Entity Input Switch/7
  MATLAB Discrete-Event System9/1 -> Subsystem6/3(In3)
  In2/1 -> Entity Replicator/1
  MATLAB Discrete-Event System1/2 -> Subsystem1/1(In1)
  Subsystem3/2(Out3) -> MATLAB Discrete-Event System8/4
  Subsystem2/1(Out1) -> Entity Input Switch/5
  MATLAB Discrete-Event System1/3 -> Subsystem2/1(In1)
  MATLAB Discrete-Event System9/3 -> Subsystem4/3(In3)
  Subsystem1/1(Out1) -> Entity Input Switch/6
  Entity Replicator/5 -> Subsystem2/2(In2)
  In1/1 -> MATLAB Discrete-Event System1/1
  MATLAB Discrete-Event System1/1 -> Subsystem/1(In1)
  Subsystem4/2(Out3) -> MATLAB Discrete-Event System8/5
  Subsystem4/1(Out1) -> Entity Input Switch/3
  MATLAB Discrete-Event System9/4 -> Subsystem3/3(In3)
  MATLAB Discrete-Event System1/4 -> Subsystem3/1(In1)
  MATLAB Discrete-Event System1/6 -> Subsystem5/1(In1)
  Entity Input Switch/1 -> Out1/1
  Subsystem/2(Out3) -> MATLAB Discrete-Event System8/1
  Subsystem3/1(Out1) -> Entity Input Switch/4
  Multicast Receive Queue/1 -> MATLAB Discrete-Event System9/1
  MATLAB Discrete-Event System9/7 -> Subsystem/3(In3)
  MATLAB Discrete-Event System1/5 -> Subsystem4/1(In1)
  Entity Replicator/4 -> Subsystem3/2(In2)
  MATLAB Discrete-Event System9/5 -> Subsystem2/3(In3)
  Subsystem2/2(Out3) -> MATLAB Discrete-Event System8/3
  Entity Replicator/3 -> Subsystem4/2(In2)
  Entity Replicator/6 -> Subsystem1/2(In2)
  Entity Replicator/1 -> Subsystem6/2(In2)
  Entity Replicator/2 -> Subsystem5/2(In2)
  Entity Replicator/7 -> Subsystem/2(In2)

== system VANETlib/Vehicle_multiChannel/Subsystem2 ==
  In1 : Inport
  MATLAB Discrete-Event System2 : MATLABDiscreteEventSystem  InputPortMessageModes=m  OutputPortMessageModes=m,m  System=des_APP_WME  vehicleID=vehicleID  enCCHIext=0  SimulateUsing=Code generation
      mask Type: des_APP_WME
      mask Display: disp('des_APP_WME');
  Out1 : Outport  VectorParamsAs1DForOutWhenUnconnected=off
  Out2 : Outport  Port=2  VectorParamsAs1DForOutWhenUnconnected=off
  wires:
  MATLAB Discrete-Event System2/1 -> Out1/1
  MATLAB Discrete-Event System2/2 -> Out2/1
  In1/1 -> MATLAB Discrete-Event System2/1

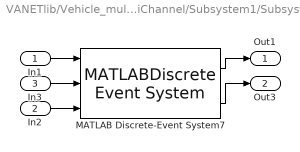
== system VANETlib/Vehicle_multiChannel/Subsystem1/Subsystem ==
  In1 : Inport
  In2 : Inport  Port=2
  In3 : Inport  Port=3
  MATLAB Discrete-Event System7 : MATLABDiscreteEventSystem  InputPortMessageModes=m,m,m  OutputPortMessageModes=m,m  System=des_MAC_mulChan_OBU  Retry_MAX=3  AIFSN_AC0=9  AIFSN_AC1=6  AIFSN_AC2=3  AIFSN_AC3=2  aCWmin=15  aCWmax=1023  slottime=13  sifs=32  txAddr=txAddr  infraAddress=0  ChanNum=chanNum  SimulateUsing=Code generation
      mask Type: des_MAC_mulChan_OBU
      mask Display: disp('des_MAC_mulChan_OBU');
  Out1 : Outport  VectorParamsAs1DForOutWhenUnconnected=off
  Out3 : Outport  Port=2  VectorParamsAs1DForOutWhenUnconnected=off
  wires:
  In2/1 -> MATLAB Discrete-Event System7/3
  In3/1 -> MATLAB Discrete-Event System7/2
  MATLAB Discrete-Event System7/1 -> Out1/1
  MATLAB Discrete-Event System7/2 -> Out3/1
  In1/1 -> MATLAB Discrete-Event System7/1

== system VANETlib/Vehicle_multiChannel/Subsystem1/Subsystem1 ==
  In1 : Inport
  In2 : Inport  Port=2
  In3 : Inport  Port=3
  MATLAB Discrete-Event System6 : MATLABDiscreteEventSystem  InputPortMessageModes=m,m,m  OutputPortMessageModes=m,m  System=des_MAC_mulChan_OBU  Retry_MAX=3  AIFSN_AC0=9  AIFSN_AC1=6  AIFSN_AC2=3  AIFSN_AC3=2  aCWmin=15  aCWmax=1023  slottime=13  sifs=32  txAddr=txAddr  infraAddress=0  ChanNum=chanNum  SimulateUsing=Code generation
      mask Type: des_MAC_mulChan_OBU
      mask Display: disp('des_MAC_mulChan_OBU');
  Out1 : Outport  VectorParamsAs1DForOutWhenUnconnected=off
  Out3 : Outport  Port=2  VectorParamsAs1DForOutWhenUnconnected=off
  wires:
  In3/1 -> MATLAB Discrete-Event System6/2
  MATLAB Discrete-Event System6/2 -> Out3/1
  In1/1 -> MATLAB Discrete-Event System6/1
  MATLAB Discrete-Event System6/1 -> Out1/1
  In2/1 -> MATLAB Discrete-Event System6/3

== system VANETlib/Vehicle_multiChannel/Subsystem1/Subsystem2 ==
  In1 : Inport
  In2 : Inport  Port=2
  In3 : Inport  Port=3
  MATLAB Discrete-Event System5 : MATLABDiscreteEventSystem  InputPortMessageModes=m,m,m  OutputPortMessageModes=m,m  System=des_MAC_mulChan_OBU  Retry_MAX=3  AIFSN_AC0=9  AIFSN_AC1=6  AIFSN_AC2=3  AIFSN_AC3=2  aCWmin=15  aCWmax=1023  slottime=13  sifs=32  txAddr=txAddr  infraAddress=0  ChanNum=chanNum  SimulateUsing=Code generation
      mask Type: des_MAC_mulChan_OBU
      mask Display: disp('des_MAC_mulChan_OBU');
  Out1 : Outport  VectorParamsAs1DForOutWhenUnconnected=off
  Out3 : Outport  Port=2  VectorParamsAs1DForOutWhenUnconnected=off
  wires:
  In1/1 -> MATLAB Discrete-Event System5/1
  MATLAB Discrete-Event System5/2 -> Out3/1
  In3/1 -> MATLAB Discrete-Event System5/2
  MATLAB Discrete-Event System5/1 -> Out1/1
  In2/1 -> MATLAB Discrete-Event System5/3

== system VANETlib/Vehicle_multiChannel/Subsystem1/Subsystem3 ==
  In1 : Inport
  In2 : Inport  Port=2
  In3 : Inport  Port=3
  MATLAB Discrete-Event System4 : MATLABDiscreteEventSystem  InputPortMessageModes=m,m,m  OutputPortMessageModes=m,m  System=des_MAC_mulChan_OBU  Retry_MAX=3  AIFSN_AC0=9  AIFSN_AC1=6  AIFSN_AC2=3  AIFSN_AC3=2  aCWmin=15  aCWmax=1023  slottime=13  sifs=32  txAddr=txAddr  infraAddress=0  ChanNum=chanNum  SimulateUsing=Code generation
      mask Type: des_MAC_mulChan_OBU
      mask Display: disp('des_MAC_mulChan_OBU');
  Out1 : Outport  VectorParamsAs1DForOutWhenUnconnected=off
  Out3 : Outport  Port=2  VectorParamsAs1DForOutWhenUnconnected=off
  wires:
  MATLAB Discrete-Event System4/1 -> Out1/1
  MATLAB Discrete-Event System4/2 -> Out3/1
  In1/1 -> MATLAB Discrete-Event System4/1
  In3/1 -> MATLAB Discrete-Event System4/2
  In2/1 -> MATLAB Discrete-Event System4/3

== system VANETlib/Vehicle_multiChannel/Subsystem1/Subsystem4 ==
  In1 : Inport
  In2 : Inport  Port=2
  In3 : Inport  Port=3
  MATLAB Discrete-Event System3 : MATLABDiscreteEventSystem  InputPortMessageModes=m,m,m  OutputPortMessageModes=m,m  System=des_MAC_mulChan_OBU  Retry_MAX=3  AIFSN_AC0=9  AIFSN_AC1=6  AIFSN_AC2=3  AIFSN_AC3=2  aCWmin=15  aCWmax=1023  slottime=13  sifs=32  txAddr=txAddr  infraAddress=0  ChanNum=chanNum  SimulateUsing=Code generation
      mask Type: des_MAC_mulChan_OBU
      mask Display: disp('des_MAC_mulChan_OBU');
  Out1 : Outport  VectorParamsAs1DForOutWhenUnconnected=off
  Out3 : Outport  Port=2  VectorParamsAs1DForOutWhenUnconnected=off
  wires:
  In3/1 -> MATLAB Discrete-Event System3/2
  In2/1 -> MATLAB Discrete-Event System3/3
  MATLAB Discrete-Event System3/1 -> Out1/1
  In1/1 -> MATLAB Discrete-Event System3/1
  MATLAB Discrete-Event System3/2 -> Out3/1

== system VANETlib/Vehicle_multiChannel/Subsystem1/Subsystem5 ==
  In1 : Inport
  In2 : Inport  Port=2
  In3 : Inport  Port=3
  MATLAB Discrete-Event System2 : MATLABDiscreteEventSystem  InputPortMessageModes=m,m,m  OutputPortMessageModes=m,m  System=des_MAC_mulChan_OBU  Retry_MAX=3  AIFSN_AC0=9  AIFSN_AC1=6  AIFSN_AC2=3  AIFSN_AC3=2  aCWmin=15  aCWmax=1023  slottime=13  sifs=32  txAddr=txAddr  infraAddress=0  ChanNum=chanNum  SimulateUsing=Code generation
      mask Type: des_MAC_mulChan_OBU
      mask Display: disp('des_MAC_mulChan_OBU');
  Out1 : Outport  VectorParamsAs1DForOutWhenUnconnected=off
  Out3 : Outport  Port=2  VectorParamsAs1DForOutWhenUnconnected=off
  wires:
  MATLAB Discrete-Event System2/2 -> Out3/1
  In2/1 -> MATLAB Discrete-Event System2/3
  In3/1 -> MATLAB Discrete-Event System2/2
  MATLAB Discrete-Event System2/1 -> Out1/1
  In1/1 -> MATLAB Discrete-Event System2/1

== system VANETlib/Vehicle_multiChannel/Subsystem1/Subsystem6 ==
  In1 : Inport
  In2 : Inport  Port=2
  In3 : Inport  Port=3
  MATLAB Discrete-Event System : MATLABDiscreteEventSystem  InputPortMessageModes=m,m,m  OutputPortMessageModes=m,m  System=des_MAC_mulChan_OBU  Retry_MAX=3  AIFSN_AC0=9  AIFSN_AC1=6  AIFSN_AC2=3  AIFSN_AC3=2  aCWmin=15  aCWmax=1023  slottime=13  sifs=32  txAddr=txAddr  infraAddress=0  ChanNum=chanNum  SimulateUsing=Code generation
      mask Type: des_MAC_mulChan_OBU
      mask Display: disp('des_MAC_mulChan_OBU');
  Out1 : Outport  VectorParamsAs1DForOutWhenUnconnected=off
  Out3 : Outport  Port=2  VectorParamsAs1DForOutWhenUnconnected=off
  wires:
  MATLAB Discrete-Event System/2 -> Out3/1
  In3/1 -> MATLAB Discrete-Event System/2
  In1/1 -> MATLAB Discrete-Event System/1
  In2/1 -> MATLAB Discrete-Event System/3
  MATLAB Discrete-Event System/1 -> Out1/1
